simulink model "RLSim2"  (R2015b)
settings: Solver=ode45  StartTime=0.0  StopTime=40*365  MaxStep=1  RelTol=1e-3
libraries: simulink x2
settings Model: Creator=jeff  LastModifiedBy=jeff
settings SolverCC: ZeroCrossAlgorithm=Adaptive
settings DataIOCC: SaveFormat=Array
settings DebuggingCC: IgnoredZcDiagnostic=none  SolverPrmCheckMsg=warning
settings HardwareCC: ProdBitPerPointer=32  ProdLargestAtomicFloat=None  ProdIntDivRoundTo=Undefined  ProdEndianess=Unspecified  ProdWordSize=32  ProdHWDeviceType=32-bit Generic
settings GRTTargetCC: GeneratePreprocessorConditionals=Disable all
settings ConfigComp: CovModelRefEnable=Off  CovSFcnEnable=off

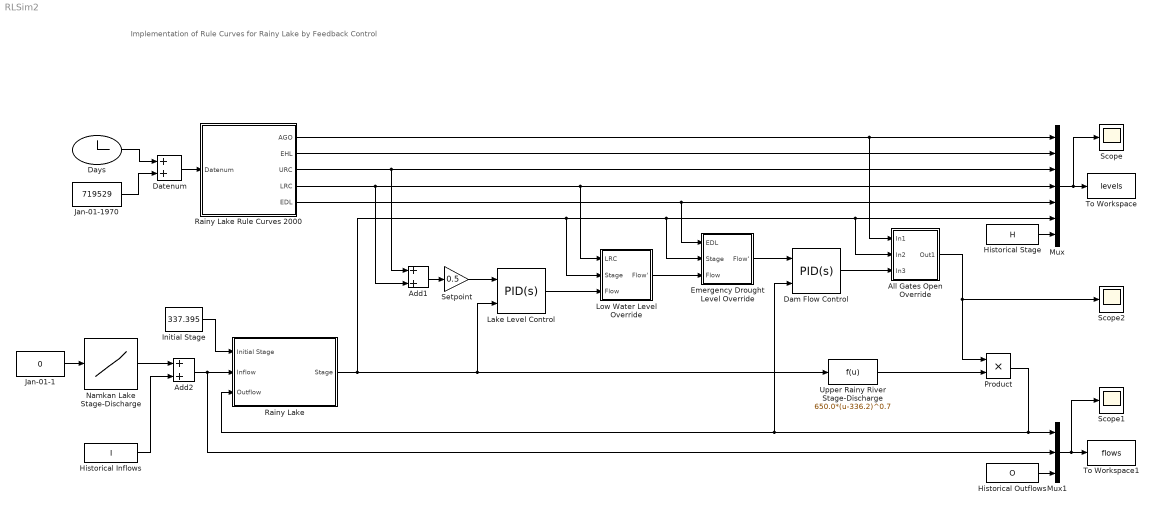
== system RLSim2 ==
  note: Implementation of Rule Curves for Rainy Lake by Feedback Control
  Add1 : Sum
  Add2 : Sum
  All Gates Open Override : Subsystem
  Dam Flow Control : simulink/Continuous/PID Controller (2DOF)  Controller=PID  TimeDomain=Continuous-time  SampleTime=-1  IntegratorMethod=Forward Euler  FilterMethod=Forward Euler  Form=Parallel  UseFilter=on  ControllerParametersSource=internal  P=0  I=0.00566146868750982  D=0  N=100  b=1  c=1  InitialConditionSource=internal  InitialConditionForIntegrator=0  InitialConditionForFilter=0  ExternalReset=none  LimitOutput=on  UpperSaturationLimit=1  LowerSaturationLimit=0  LinearizeAsGain=off  AntiWindupMode=clamping  Kb=1  TrackingMode=off  Kt=1  PParamMin=[]  PParamMax=[]  IParamMin=[]  IParamMax=[]  DParamMin=[]  DParamMax=[]  NParamMin=[]  NParamMax=[]  bParamMin=[]  bParamMax=[]  cParamMin=[]  cParamMax=[]  KbParamMin=[]  KbParamMax=[]  KtParamMin=[]  KtParamMax=[]  POutMin=[]  POutMax=[]  IOutMin=[]  IOutMax=[]  DOutMin=[]  DOutMax=[]  NOutMin=[]  NOutMax=[]  bOutMin=[]  bOutMax=[]  cOutMin=[]  cOutMax=[]  KbOutMin=[]  KbOutMax=[]  KtOutMin=[]  KtOutMax=[]  IntegratorOutMin=[]  IntegratorOutMax=[]  FilterOutMin=[]  FilterOutMax=[]  SumOutMin=[]  SumOutMax=[]  Sum1OutMin=[]  Sum1OutMax=[]  Sum2OutMin=[]  Sum2OutMax=[]  Sum3OutMin=[]  Sum3OutMax=[]  SumI1OutMin=[]  SumI1OutMax=[]  SumI2OutMin=[]  SumI2OutMax=[]  SumI3OutMin=[]  SumI3OutMax=[]  SumDOutMin=[]  SumDOutMax=[]  SaturationOutMin=[]  SaturationOutMax=[]  IntegratorContinuousStateAttributes=''  IntegratorStateMustResolveToSignalObject=off  IntegratorRTWStateStorageClass=Auto  FilterContinuousStateAttributes=''  FilterStateMustResolveToSignalObject=off  FilterRTWStateStorageClass=Auto  DifferentiatorICPrevScaledInput=0  DifferentiatorOutMin=[]  DifferentiatorOutMax=[]
  Datenum : Sum
  Days : Clock
  Emergency Drought Level Override : Subsystem
  Historical Inflows : FromWorkspace  VariableName=I  SampleTime=1
  Historical Outflows : FromWorkspace  VariableName=O  SampleTime=1
  Historical Stage : FromWorkspace  VariableName=H  SampleTime=1
  Initial Stage : Constant  Value=337.395
  Jan-01-1 : Constant  Value=0
  Jan-01-1970 : Constant  Value=719529
  Lake Level Control : simulink/Continuous/PID Controller (2DOF)  Controller=PID  TimeDomain=Continuous-time  SampleTime=-1  IntegratorMethod=Forward Euler  FilterMethod=Forward Euler  Form=Ideal  UseFilter=on  ControllerParametersSource=internal  P=-200  I=0.96903600242824  D=0.18000786280984  N=27.0758760802227  b=0.549490026184705  c=0.0103938234350511  InitialConditionSource=internal  InitialConditionForIntegrator=0  InitialConditionForFilter=0  ExternalReset=none  LimitOutput=on  UpperSaturationLimit=2000  LowerSaturationLimit=100  LinearizeAsGain=off  AntiWindupMode=clamping  Kb=1  TrackingMode=off  Kt=1  PParamMin=[]  PParamMax=[]  IParamMin=[]  IParamMax=[]  DParamMin=[]  DParamMax=[]  NParamMin=[]  NParamMax=[]  bParamMin=[]  bParamMax=[]  cParamMin=[]  cParamMax=[]  KbParamMin=[]  KbParamMax=[]  KtParamMin=[]  KtParamMax=[]  POutMin=[]  POutMax=[]  IOutMin=[]  IOutMax=[]  DOutMin=[]  DOutMax=[]  NOutMin=[]  NOutMax=[]  bOutMin=[]  bOutMax=[]  cOutMin=[]  cOutMax=[]  KbOutMin=[]  KbOutMax=[]  KtOutMin=[]  KtOutMax=[]  IntegratorOutMin=[]  IntegratorOutMax=[]  FilterOutMin=[]  FilterOutMax=[]  SumOutMin=[]  SumOutMax=[]  Sum1OutMin=[]  Sum1OutMax=[]  Sum2OutMin=[]  Sum2OutMax=[]  Sum3OutMin=[]  Sum3OutMax=[]  SumI1OutMin=[]  SumI1OutMax=[]  SumI2OutMin=[]  SumI2OutMax=[]  SumI3OutMin=[]  SumI3OutMax=[]  SumDOutMin=[]  SumDOutMax=[]  SaturationOutMin=[]  SaturationOutMax=[]  IntegratorContinuousStateAttributes=''  IntegratorStateMustResolveToSignalObject=off  IntegratorRTWStateStorageClass=Auto  FilterContinuousStateAttributes=''  FilterStateMustResolveToSignalObject=off  FilterRTWStateStorageClass=Auto  DifferentiatorICPrevScaledInput=0  DifferentiatorOutMin=[]  DifferentiatorOutMax=[]
  Low Water Level Override : Subsystem
  Mux : Mux  Inputs=7
  Mux1 : Mux  Inputs=3
  Namkan Lake Stage-Discharge : Lookup_n-D  NumberOfTableDimensions=1  BreakpointsForDimension1=[335.21, 337.0, 338.0, 338.5, 339.0, 339.5, 340.0, 340.5, 341.0, 341.5, 342.0, 342.5, 343.0]  Table=[0 51 120 173 233 299 373 455 549 659 772 886 999]  ExtrapMethod=Clip  InternalRulePriority=Speed  RndMeth=Simplest  InputSameDT=on
  Product : Product
  Rainy Lake : Subsystem
  Rainy Lake Rule Curves 2000 : Subsystem
  Scope : Scope
  Scope1 : Scope
  Scope2 : Scope
  Setpoint : Gain  Gain=0.5
  To Workspace : ToWorkspace  VariableName=levels  SaveFormat=Timeseries  SampleTime=-1
  To Workspace1 : ToWorkspace  VariableName=flows  SaveFormat=Timeseries  SampleTime=-1
  Upper Rainy River Stage-Discharge : Fcn  Expr=650.0*(u-336.2)^0.7
  wires:
  Days/1 -> Datenum/1
  Jan-01-1970/1 -> Datenum/2
  Datenum/1 -> Rainy Lake Rule Curves 2000/1(Datenum)
  Mux/1 -> Scope/1, To Workspace/1
  Add1/1 -> Setpoint/1
  Setpoint/1 -> Lake Level Control/1
  Rainy Lake Rule Curves 2000/3(URC) -> Mux/3, Add1/1
  Rainy Lake Rule Curves 2000/4(LRC) -> Mux/4, Low Water Level Override/1(LRC), Add1/2
  Initial Stage/1 -> Rainy Lake/1(Initial Stage)
  Mux1/1 -> Scope1/1, To Workspace1/1
  Rainy Lake Rule Curves 2000/1(AGO) -> Mux/1, All Gates Open Override/1(In1)
  Historical Stage/1 -> Mux/7
  Historical Outflows/1 -> Mux1/3
  Rainy Lake Rule Curves 2000/2(EHL) -> Mux/2
  Add2/1 -> Mux1/2, Rainy Lake/2(Inflow)
  Namkan Lake Stage-Discharge/1 -> Add2/1
  Historical Inflows/1 -> Add2/2
  Jan-01-1/1 -> Namkan Lake Stage-Discharge/1
  Upper Rainy River Stage-Discharge/1 -> Product/2
  Product/1 -> Rainy Lake/3(Outflow), Dam Flow Control/2, Mux1/1
  Rainy Lake Rule Curves 2000/5(EDL) -> Mux/5, Emergency Drought Level Override/1(EDL)
  Rainy Lake/1(Stage) -> Mux/6, All Gates Open Override/2(In2), Emergency Drought Level Override/2(Stage), Low Water Level Override/2(Stage), Upper Rainy River Stage-Discharge/1, Lake Level Control/2
  Lake Level Control/1 -> Low Water Level Override/3(Flow)
  Low Water Level Override/1(Flow') -> Emergency Drought Level Override/3(Flow)
  Emergency Drought Level Override/1(Flow') -> Dam Flow Control/1
  Dam Flow Control/1 -> All Gates Open Override/3(In3)
  All Gates Open Override/1(Out1) -> Product/1, Scope2/1

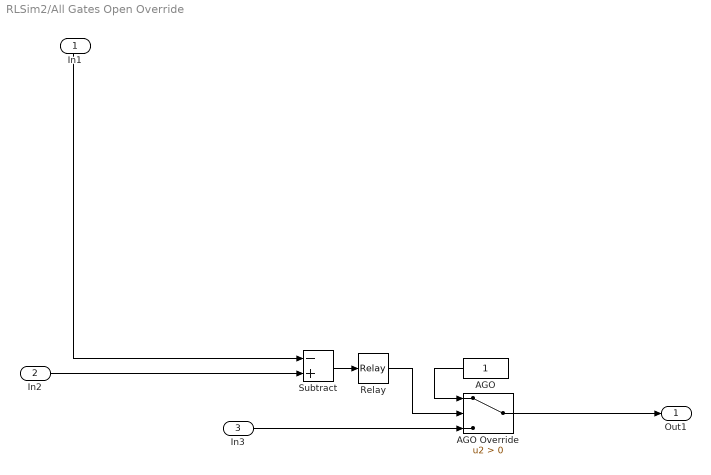
== system RLSim2/All Gates Open Override ==
  In1 : Inport
  In2 : Inport  Port=2
  In3 : Inport  Port=3
  AGO : Constant
  AGO Override : Switch  Criteria=u2 > Threshold
  Relay : Relay  OnSwitchValue=0.02  OffSwitchValue=-0.02
  Subtract : Sum  Inputs=-+
  Out1 : Outport
  wires:
  Relay/1 -> AGO Override/2
  In3/1 -> AGO Override/3
  Subtract/1 -> Relay/1
  In2/1 -> Subtract/2
  AGO/1 -> AGO Override/1
  AGO Override/1 -> Out1/1
  In1/1 -> Subtract/1

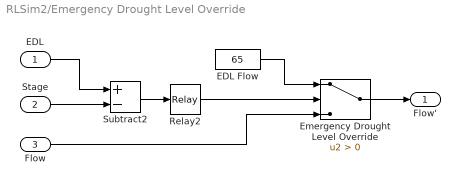
== system RLSim2/Emergency Drought Level Override ==
  EDL : Inport
  Stage : Inport  Port=2
  Flow : Inport  Port=3
  EDL Flow : Constant  Value=65
  Emergency Drought Level Override : Switch  Criteria=u2 > Threshold
  Relay2 : Relay  OnSwitchValue=0.02  OffSwitchValue=-0.02
  Subtract2 : Sum  Inputs=+-
  Flow' : Outport
  wires:
  Subtract2/1 -> Relay2/1
  Stage/1 -> Subtract2/2
  Emergency Drought Level Override/1 -> Flow'/1
  EDL Flow/1 -> Emergency Drought Level Override/1
  EDL/1 -> Subtract2/1
  Relay2/1 -> Emergency Drought Level Override/2
  Flow/1 -> Emergency Drought Level Override/3

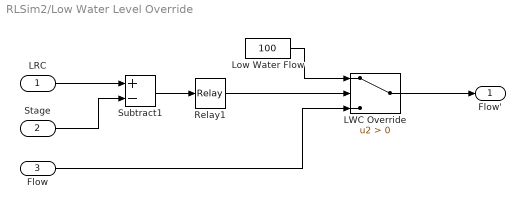
== system RLSim2/Low Water Level Override ==
  LRC : Inport
  Stage : Inport  Port=2
  Flow : Inport  Port=3
  LWC Override : Switch  Criteria=u2 > Threshold
  Low Water Flow : Constant  Value=100
  Relay1 : Relay  OnSwitchValue=0.02  OffSwitchValue=-0.02
  Subtract1 : Sum  Inputs=+-
  Flow' : Outport
  wires:
  Relay1/1 -> LWC Override/2
  Low Water Flow/1 -> LWC Override/1
  LWC Override/1 -> Flow'/1
  Subtract1/1 -> Relay1/1
  Flow/1 -> LWC Override/3
  LRC/1 -> Subtract1/1
  Stage/1 -> Subtract1/2

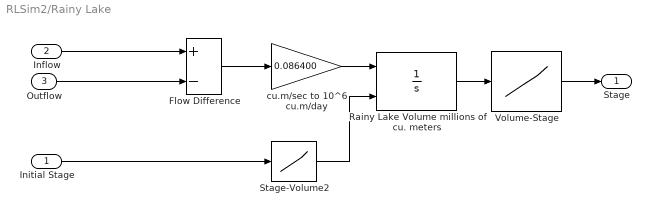
== system RLSim2/Rainy Lake ==
  Initial Stage : Inport
  Inflow : Inport  Port=2
  Outflow : Inport  Port=3
  Flow Difference : Sum  Inputs=+-
  Rainy Lake Volume millions of cu. meters : Integrator  InitialConditionSource=external  InitialCondition=1000  LimitOutput=on  LowerSaturationLimit=0  ContinuousStateAttributes='RainyLakeVolume'
  Stage-Volume2 : Lookup_n-D  NumberOfTableDimensions=1  BreakpointsForDimension1=[335.0 336.0 336.5 337.0 337.5 338.0 339.0 340.0]  Table=[112.67 798.00 1176.42 1577.25 2002.06 2450.57 3416.85 4458.97]  InternalRulePriority=Speed  RndMeth=Simplest  InputSameDT=on
  Volume-Stage : Lookup_n-D  NumberOfTableDimensions=1  BreakpointsForDimension1=[112.67 798.00 1176.42 1577.25 2002.06 2450.57 3416.85 4458.97]  Table=[335.0 336.0 336.5 337.0 337.5 338.0 339.0 340.0]  InternalRulePriority=Speed  RndMeth=Simplest  InputSameDT=on
  cu.m/sec to 10^6 cu.m/day : Gain  Gain=0.086400
  Stage : Outport
  wires:
  Outflow/1 -> Flow Difference/2
  Inflow/1 -> Flow Difference/1
  Rainy Lake Volume millions of cu. meters/1 -> Volume-Stage/1
  Stage-Volume2/1 -> Rainy Lake Volume millions of cu. meters/2
  cu.m/sec to 10^6 cu.m/day/1 -> Rainy Lake Volume millions of cu. meters/1
  Initial Stage/1 -> Stage-Volume2/1
  Volume-Stage/1 -> Stage/1
  Flow Difference/1 -> cu.m/sec to 10^6 cu.m/day/1

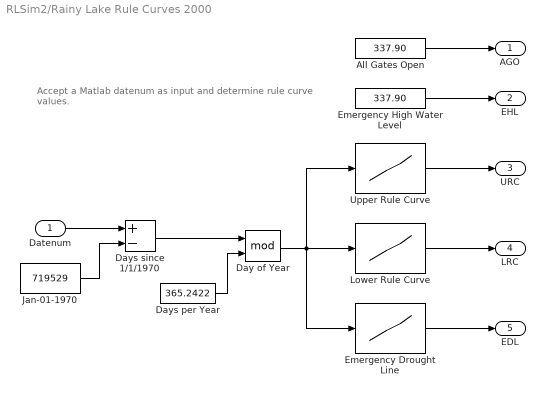
== system RLSim2/Rainy Lake Rule Curves 2000 ==
  note: Accept a Matlab datenum as input and determine rule curve values.
  Datenum : Inport
  All Gates Open : Constant  Value=337.90
  Day of Year : Math  Operator=mod  SaturateOnIntegerOverflow=on
  Days per Year : Constant  Value=365.2422
  Days since 1/1/1970 : Sum  Inputs=+-
  Emergency Drought Line : Lookup_n-D  NumberOfTableDimensions=1  BreakpointsForDimension1=[0 91 181 182 297 366]  Table=[336.90 336.70 336.70 337.20 337.20 336.90]  InternalRulePriority=Speed  RndMeth=Simplest  InputSameDT=on
  Emergency High Water Level : Constant  Value=337.90
  Jan-01-1970 : Constant  Value=719529
  Lower Rule Curve : Lookup_n-D  NumberOfTableDimensions=1  BreakpointsForDimension1=[0 91 121 152 182 227 335 366]  Table=[337.20 336.70 336.80 337.30 337.50 337.50 337.30 337.20]  InternalRulePriority=Speed  RndMeth=Simplest  InputSameDT=on
  Upper Rule Curve : Lookup_n-D  NumberOfTableDimensions=1  BreakpointsForDimension1=[0 91 121 152 182 227 335 366]  Table="[337.45 337.0  337.40 337.60 337.75 337.75 337.60 337.45]"  InternalRulePriority=Speed  RndMeth=Simplest  InputSameDT=on
  AGO : Outport
  EHL : Outport  Port=2
  URC : Outport  Port=3
  LRC : Outport  Port=4
  EDL : Outport  Port=5
  wires:
  Jan-01-1970/1 -> Days since 1/1/1970/2
  Days since 1/1/1970/1 -> Day of Year/1
  Days per Year/1 -> Day of Year/2
  Day of Year/1 -> Upper Rule Curve/1, Emergency Drought Line/1, Lower Rule Curve/1
  Upper Rule Curve/1 -> URC/1
  Lower Rule Curve/1 -> LRC/1
  Datenum/1 -> Days since 1/1/1970/1
  All Gates Open/1 -> AGO/1
  Emergency Drought Line/1 -> EDL/1
  Emergency High Water Level/1 -> EHL/1
